simulink model "inverted_pendulum_on_cart2016"  (R2016a)
settings: Solver=VariableStepAuto  SolverMode=SingleTasking  StartTime=0.0  StopTime=10.0  RelTol=1e-3
values from neighbouring files (symbols this model uses):
  b = 0.1    [Inverted_pendulum_on_cart.mat]
  g = 9.8    [Inverted_pendulum_on_cart.mat]
  l = 0.3    [Inverted_pendulum_on_cart.mat]
  M = 0.5    [Inverted_pendulum_on_cart.mat]
  m = 0.2    [Inverted_pendulum_on_cart.mat]
undefined symbols (not defined in the file or in its folder): i
settings Model: Creator=Ranish  LastModifiedBy=Ranish
settings DataIOCC: ReturnWorkspaceOutputs=on
settings DebuggingCC: SFUnexpectedBacktrackingDiag=error  SFNoUnconditionalDefaultTransitionDiag=error
settings SFSimCC: SimUseLocalCustomCode=on
settings RTWCC: RTWUseLocalCustomCode=on
settings GRTTargetCC: TargetLangStandard=C99 (ISO)  GeneratePreprocessorConditionals=Use local settings
settings ConfigComp: CovMetricSettings=dwe  CovHtmlReporting=off  CovSaveCumulativeToWorkspaceVar=off  CovSaveSingleToWorkspaceVar=off  CovExternalEMLEnable=on

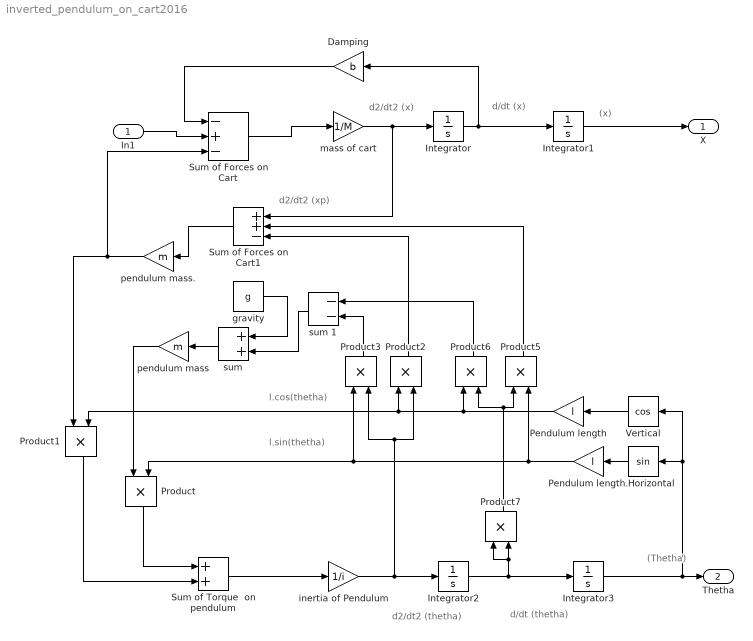
== system inverted_pendulum_on_cart2016 ==
  note: l.cos(thetha)
  note: (Thetha)
  note: (x)
  note: d/dt (thetha)
  note: d2/dt2 (thetha)
  note: d/dt (x)
  note: d2/dt2 (x)
  note: d2/dt2 (xp)
  note: l.sin(thetha)
  In1 : Inport
  Damping : Gain  Gain=b
  Horizontal : Trigonometry
  Integrator{,1..3} (4 alike) : Integrator
  Pendulum length : Gain  Gain=l
  Pendulum length. : Gain  Gain=l
  Product{,1..3,5..7} (7 alike) : Product
  Sum of Forces on Cart : Sum  Inputs=-+-
  Sum of Forces on Cart1 : Sum  Inputs=++-
  Sum of Torque  on pendulum : Sum
  Vertical : Trigonometry  Operator=cos
  gravity : Constant  Value=g
  "inertia of Pendulum " : Gain  Gain=1/i
  mass of cart : Gain  Gain=1/M
  "pendulum mass " : Gain  Gain=m
  "pendulum mass. " : Gain  Gain=m
  "sum " : Sum
  sum 1 : Sum  Inputs=--
  "X " : Outport
  "Thetha " : Outport  Port=2
  wires:
  Sum of Forces on Cart/1 -> mass of cart/1
  mass of cart/1 -> Sum of Forces on Cart1/1, Integrator/1
  Integrator/1 -> Damping/1, Integrator1/1
  Integrator2/1 -> Integrator3/1, Product7/1, Product7/2
  "inertia of Pendulum "/1 -> Integrator2/1, Product3/2, Product2/2
  Sum of Torque  on pendulum/1 -> "inertia of Pendulum "/1
  Damping/1 -> Sum of Forces on Cart/1
  In1/1 -> Sum of Forces on Cart/2
  Integrator3/1 -> "Thetha "/1, Horizontal/1, Vertical/1
  Integrator1/1 -> "X "/1
  Horizontal/1 -> Pendulum length./1
  Vertical/1 -> Pendulum length/1
  Product/1 -> Sum of Torque  on pendulum/1
  Product1/1 -> Sum of Torque  on pendulum/2
  Pendulum length./1 -> Product3/1, Product/2, Product5/2
  Pendulum length/1 -> Product2/1, Product1/2, Product6/1
  "pendulum mass "/1 -> Product/1
  "pendulum mass. "/1 -> Sum of Forces on Cart/3, Product1/1
  "sum "/1 -> "pendulum mass "/1
  gravity/1 -> "sum "/1
  sum 1/1 -> "sum "/2
  Sum of Forces on Cart1/1 -> "pendulum mass. "/1
  Product7/1 -> Product5/1, Product6/2
  Product5/1 -> Sum of Forces on Cart1/2
  Product2/1 -> Sum of Forces on Cart1/3
  Product6/1 -> sum 1/1
  Product3/1 -> sum 1/2
